simulink model "vdn7_planning_trace_MPC"  (R2022b)
settings: Solver=ode45  StartTime=0.0  StopTime=40  FixedStep=0.01  RelTol=1e-3  EnableMultiTasking=on
libraries: Solver_SF x1
settings Model: Creator=xuwei  LastModifiedBy=wyx
settings SolverCC: AlgebraicLoopSolver=TrustRegion
settings DataIOCC: LimitDataPoints=on  SaveFormat=Array  SignalLoggingSaveFormat=ModelDataLogs  ReturnWorkspaceOutputs=off
settings OptimizationCC: ExpressionDepthLimit=2147483647  LifeSpan=inf
settings DebuggingCC: UnderspecifiedInitializationDetection=Classic  MergeDetectMultiDrivingBlocksExec=none  SolverPrmCheckMsg=warning  FcnCallInpInsideContextMsg=warning  UnconnectedInputMsg=warning  UnconnectedOutputMsg=warning  UnconnectedLineMsg=warning  StateNameClashWarn=warning  SFUnexpectedBacktrackingDiag=warning  SFNoUnconditionalDefaultTransitionDiag=warning  SFExecutionAtInitializationDiag=none  SFMachineParentedDataDiag=warning  ArithmeticOperatorsInVariantConditions=warning
settings HardwareCC: ProdBitPerPointer=32  ProdBitPerSizeT=32  ProdBitPerPtrDiffT=32  ProdLargestAtomicFloat=None  ProdIntDivRoundTo=Undefined  ProdEndianess=Unspecified  ProdWordSize=32  ProdHWDeviceType=32-bit Generic
settings ModelReferenceCC: PropagateSignalLabelsOutOfModel=off
settings SFSimCC: SimUseLocalCustomCode=off  CustomCodeUndefinedFunction=UseInterfaceOnly
settings RTWCC: RTWUseLocalCustomCode=off
settings CodeAppCC: StateflowObjectComments=on
settings GRTTargetCC: TargetLangStandard=C89/C90 (ANSI)  CombineOutputUpdateFcns=off  GRTInterface=on
settings ConfigComp: CovMetricSettings=dw  CovSaveCumulativeToWorkspaceVar=on  CovSaveSingleToWorkspaceVar=on  CovExternalEMLEnable=off
settings SimscapeCC: SimscapeNormalizeSystem=off
settings ConfigurationSet: Description=SimMechanics 2G

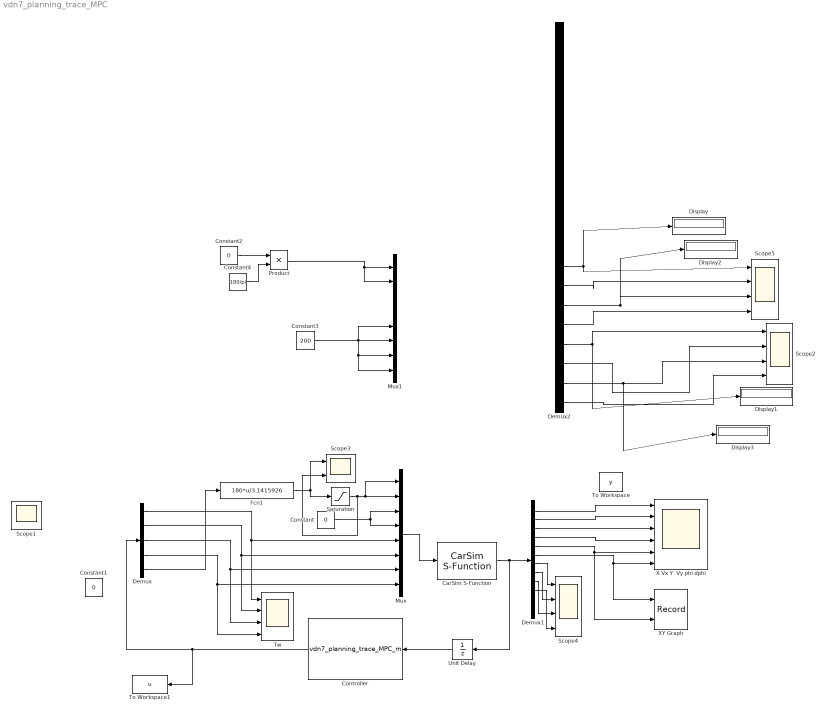
== system vdn7_planning_trace_MPC ==
  CarSim S-Function : Solver_SF/CarSim S-Function  Priority=1  SIMFILE=simfile.sim
  Constant : Constant  Value=0
  Constant1 : Constant  Value=0
  Constant2 : Constant  Value=0
  Constant3 : Constant  Value=200
  Constant4 : Constant  Value=180/pi
  Controller : S-Function  FunctionName=vdn7_planning_trace_MPC_m  SFunctionDeploymentMode=off  EnableBusSupport=off
  Demux : Demux  Outputs=5
  Demux1 : Demux  Outputs=12
  Demux2 : Demux  Outputs=20
  Display{,1..3} (4 alike) : Display
  Fcn1 : Fcn  Expr=180*u/3.1415926
  Mux : Mux  Inputs=8
  Mux1 : Mux  Inputs=8
  Product : Product
  Saturation : Saturate  UpperLimit=30  LowerLimit=-30
  Scope1 : Scope  NumInputPorts=2
  Scope2 : Scope  NumInputPorts=4
  Scope3 : Scope  NumInputPorts=2
  Scope4 : Scope  NumInputPorts=4
  Scope5 : Scope  NumInputPorts=4
  To Workspace : ToWorkspace  VariableName=y  SaveFormat=Structure  SampleTime=-1
  To Workspace1 : ToWorkspace  VariableName=u  SaveFormat=Structure  SampleTime=-1
  Tw : Scope  NumInputPorts=4
  Unit Delay : UnitDelay  SampleTime=-1  HasFrameUpgradeWarning=on
  X Vx Y  Vy phi dphi : Scope  NumInputPorts=6
  XY Graph : Record  FileSettingsInternal="{\"entries\":[{\"content\":{\"excelSettings\":{\"content\":{},\"type\":\"Streamout.ExcelSettings\"}},\"type\":\"Streamout.FileSettingStorage\",\"uuid\":\"61cb6f9a-6c0f-4e75-bbe9-51497279b69e\"}],\"packageUris\":[\"http://schema.mathworks.com/mf0/streamout_blocks/R2020a\"],\"version\":\"1.0\"}"  Layout=[1 1]  SignalsInternal="{\"entries\":[{\"content\":{\"signals\":[{\"content\":{\"blockPath\":[\"vdn7_planning_trace_MPC/XY Graph\"],\"channel\":[],\"dimensions\":[1],\"domain\":\"vdn7_planning_trace_MPC/XY Graph\",\"lineColor\":\"#a2142f\",\"plots\":[],\"port\":1,\"sid\":[\"\"],\"signalID\":4808,\"signalName\":\"Demux1:6\"},\"type\":\"RecordBlkView.Signal\",\"uuid\":\"b09efcec-8541-4a3a-9e30-c67ddcc85211\"},{\"content\":{\"blockPath\":[\"vdn7_planning_trace_MPC/XY Graph\"],\"channel\":[],\"dimensions\":[1],\"domain\":\"vdn7_planning_trace_MPC/XY Graph\",\"lineColor\":\"#139fff\",\"plots\":[],\"port\":2,\"sid\":[\"\"],\"signalID\":4812,\"signalName\":\"Demux1:5\"},\"type\":\"RecordBlkView.Signal\",\"uuid\":\"476ee765-7e8f-4d8e-a06b-87171ab59f67\"}]},\"type\":\"RecordBlkView.InputSignals\",\"uuid\":\"9ae3c257-f1fb-4eee-9903-79515357faab\"}],\"packageUris\":[\"http://schema.mathworks.com/mf0/streamout_blocks/R2020a\"],\"version\":\"1.0\"}"  VisualizationBindings="{\"xyplotplugin\":{\"info\":[{\"series\":[],\"subplotID\":1}]}}"  CompatibilityTag=XY  st=-1
  wires:
  Demux1/1 -> X Vx Y  Vy phi dphi/1
  Demux1/2 -> X Vx Y  Vy phi dphi/2
  Demux1/3 -> X Vx Y  Vy phi dphi/3
  Demux1/5 -> XY Graph/2, X Vx Y  Vy phi dphi/5
  Demux1/6 -> XY Graph/1, X Vx Y  Vy phi dphi/6
  Constant/1 -> Mux/3, Mux/4
  Fcn1/1 -> Scope3/1, Saturation/1
  Demux1/4 -> X Vx Y  Vy phi dphi/4
  Demux1/7 -> Scope4/1
  Demux1/8 -> Scope4/2
  Demux1/9 -> Scope4/3
  Demux1/10 -> Scope4/4
  Constant2/1 -> Product/1
  Unit Delay/1 -> Controller/1
  Saturation/1 -> Scope3/2, Mux/1, Mux/2
  Demux/2 -> Tw/2, Mux/6
  Demux/3 -> Tw/3, Mux/7
  Demux/4 -> Tw/4, Mux/8
  Demux/1 -> Mux/5, Tw/1
  Controller/1 -> To Workspace1/1, Demux/1
  Demux/5 -> Fcn1/1
  Constant3/1 -> Mux1/7, Mux1/8, Mux1/5, Mux1/6
  Demux2/17 -> Display1/1, Scope2/1
  Demux2/18 -> Scope2/2
  Demux2/19 -> Display3/1, Scope2/3
  Demux2/20 -> Scope2/4
  Demux2/13 -> Display/1, Scope5/1
  Demux2/14 -> Scope5/2
  Demux2/15 -> Display2/1, Scope5/3
  Demux2/16 -> Scope5/4
  Product/1 -> Mux1/2, Mux1/1
  Constant4/1 -> Product/2
  CarSim S-Function/1 -> Unit Delay/1, Demux1/1
  Mux/1 -> CarSim S-Function/1
